simulink model "lim_grow_matlab"  (Simulink 7.9)
settings: Solver=ode45  StartTime=0.0  StopTime=1.0  RelTol=1e-3
values from neighbouring files (symbols this model uses):
  c = 1    [lim_grow_script.m]    (also in predprey.m = 3)
  P0 = 1    [lim_grow_script.m]
  r = 10    [lim_grow_script.m]    (also in sir.m = 0.55)
settings Model: Creator=Daniel  LastModifiedBy=Daniel

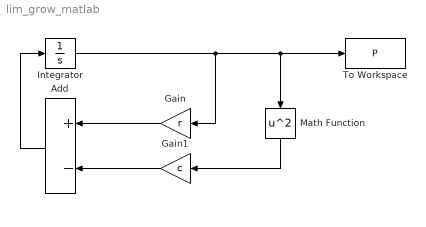
== system lim_grow_matlab ==
  Add : Sum  Inputs=+-
  Gain : Gain  Gain=r
  Gain1 : Gain  Gain=c
  Integrator : Integrator  InitialCondition=P0
  Math Function : Math  Operator=square  SaturateOnIntegerOverflow=on
  To Workspace : ToWorkspace  VariableName=P  SampleTime=-1
  wires:
  Integrator/1 -> Gain/1, Math Function/1, To Workspace/1
  Math Function/1 -> Gain1/1
  Gain/1 -> Add/1
  Gain1/1 -> Add/2
  Add/1 -> Integrator/1
